simulink model "model5"  (R2022a)
settings: Solver=VariableStepAuto  StartTime=0.0  StopTime=20  MaxStep=0.05  RelTol=1e-3  AbsTol=1e-3  EnableMultiTasking=on
PostLoadFcn:
  | m = 3.600;     % kg
  | k = 400;    % N/m
  | b = 10;      % Ns/m
CloseFcn:
  | try,close(h1_ssc_mass_spring_damper_sl_dbl),end
  | clear h1_ssc_mass_spring_damper_sl_dbl
  | 
  | clear simlog_ssc_mass_spring_damper_sl_dbl
  | clear logsout_ssc_mass_spring_damper_sl_dbl
Description:
  | Double Mass-Spring-Damper in Simulink(R) and Simscape(TM)
settings Model: Creator=The MathWorks, Inc.  LastModifiedBy=whatastarrynight
settings SolverCC: AutoScaleAbsTol=off  AlgebraicLoopSolver=TrustRegion
settings DataIOCC: LimitDataPoints=on  SaveFormat=Array  ReturnWorkspaceOutputs=off  SignalLoggingName=logsout_ssc_mass_spring_damper_sl_dbl
settings OptimizationCC: LifeSpan=inf
settings DebuggingCC: SolverPrmCheckMsg=warning  UnconnectedInputMsg=warning  UnconnectedOutputMsg=warning  UnconnectedLineMsg=warning  AllowSymbolicDim=off  PregeneratedLibrarySubsystemCodeDiagnostic=none  SFUnexpectedBacktrackingDiag=warning  SFNoUnconditionalDefaultTransitionDiag=warning  SFExecutionAtInitializationDiag=none  SFMachineParentedDataDiag=warning  ArithmeticOperatorsInVariantConditions=warning
settings HardwareCC: ProdBitPerPointer=32  ProdBitPerSizeT=32  ProdBitPerPtrDiffT=32  ProdLargestAtomicFloat=None  ProdIntDivRoundTo=Undefined  ProdEndianess=Unspecified  ProdWordSize=32  ProdHWDeviceType=32-bit Generic
settings ModelReferenceCC: PropagateSignalLabelsOutOfModel=off
settings SFSimCC: SimUseLocalCustomCode=off  CustomCodeUndefinedFunction=UseInterfaceOnly
settings RTWCC: RTWUseLocalCustomCode=off  DLArmComputeVersion=19.05
settings CodeAppCC: StateflowObjectComments=on
settings GRTTargetCC: TargetLangStandard=C89/C90 (ANSI)
settings ConfigComp: CovMetricSettings=dw  CovSaveCumulativeToWorkspaceVar=on  CovSaveSingleToWorkspaceVar=on  CovExternalEMLEnable=off  CovSFcnEnable=off
settings SimscapeCC: SimscapeLogType=all  SimscapeLogSimulationStatistics=on  SimscapeLogName=simlog_ssc_mass_spring_damper_sl_dbl  SimscapeLogDataHistory=10000

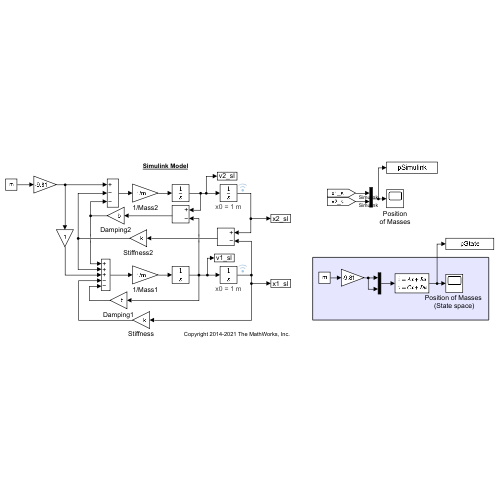
[thumbnail: Simulink's stored preview of the top-level diagram]
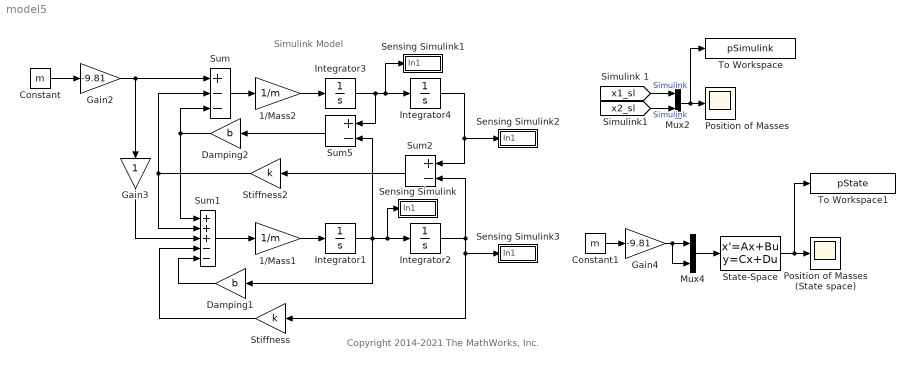
== system model5 ==
  note: Simulink Model
  note: Copyright 2014-2021 The MathWorks, Inc.
  1/Mass1 : Gain  Gain=1/m  SaturateOnIntegerOverflow=on  OutDataTypeStr=Inherit: Same as input  ParamDataTypeStr=Inherit: Same as input
  1/Mass2 : Gain  Gain=1/m  SaturateOnIntegerOverflow=on  OutDataTypeStr=Inherit: Same as input  ParamDataTypeStr=Inherit: Same as input
  Constant : Constant  Value=m
  Constant1 : Constant  Value=m
  Damping1 : Gain  Gain=b  SaturateOnIntegerOverflow=on  OutDataTypeStr=Inherit: Same as input  ParamDataTypeStr=Inherit: Same as input
  Damping2 : Gain  Gain=b  SaturateOnIntegerOverflow=on  OutDataTypeStr=Inherit: Same as input  ParamDataTypeStr=Inherit: Same as input
  Gain2 : Gain  Gain=-9.81
  Gain3 : Gain
  Gain4 : Gain  Gain=-9.81
  Integrator1 : Integrator
  Integrator2 : Integrator  InitialCondition=1
      settings: AttributesFormatString=x0 = %<InitialCondition> m
  Integrator3 : Integrator
  Integrator4 : Integrator  InitialCondition=1
      settings: AttributesFormatString=x0 = %<InitialCondition> m
  Mux2 : Mux  Inputs=2
  Mux4 : Mux  Inputs=2
  Position of Masses : Scope
  Position of Masses (State space) : Scope
  Sensing Simulink : Subsystem
      mask Display: disp('v1_sl')
  Sensing Simulink1 : Subsystem
      mask Display: disp('v2_sl')
  Sensing Simulink2 : Subsystem
      mask Display: disp('x2_sl')
  Sensing Simulink3 : Subsystem
      mask Display: disp('x1_sl')
  State-Space : StateSpace  A=[0,1,0,0;-2*k/m,-2*b/m,k/m,b/m;0,0,0,1;k/m,b/m,-k/m,-b/m]  B=[0,0;1/m,0;0,0;0,1/m]  C=[1,0,0,0;0,0,1,0]  D=[0,0;0,0]  InitialCondition=[1,0,1,0]
  Stiffness : Gain  Gain=k  SaturateOnIntegerOverflow=on  OutDataTypeStr=Inherit: Same as input  ParamDataTypeStr=Inherit: Same as input
  Stiffness2 : Gain  Gain=k  SaturateOnIntegerOverflow=on  OutDataTypeStr=Inherit: Same as input  ParamDataTypeStr=Inherit: Same as input
  Sum : Sum  Inputs=+--  InputSameDT=on  SaturateOnIntegerOverflow=on  OutDataTypeStr=Inherit: Same as first input
  Sum1 : Sum  Inputs=+++--  InputSameDT=on  SaturateOnIntegerOverflow=on  OutDataTypeStr=Inherit: Same as first input
  Sum2 : Sum  Inputs=+-  InputSameDT=on  SaturateOnIntegerOverflow=on  OutDataTypeStr=Inherit: Same as first input
  Sum5 : Sum  Inputs=+-  InputSameDT=on  SaturateOnIntegerOverflow=on  OutDataTypeStr=Inherit: Same as first input
  To Workspace : ToWorkspace  VariableName=pSimulink  SaveFormat=Timeseries  SampleTime=-1
  To Workspace1 : ToWorkspace  VariableName=pState  SaveFormat=Timeseries  SampleTime=-1
  wires:
  1/Mass1/1 -> Integrator1/1
  Sum1/1 -> 1/Mass1/1
  Sum5/1 -> Damping2/1
  Damping2/1 -> Sum1/1, Sum/3
  1/Mass2/1 -> Integrator3/1
  Sum/1 -> 1/Mass2/1
  Integrator4/1 -> Sensing Simulink2/1(In1), Sum2/1
  Integrator3/1 -> Sensing Simulink1/1(In1), Integrator4/1, Sum5/1
  Sum2/1 -> Stiffness2/1
  Stiffness2/1 -> Sum1/2, Sum/2
  Damping1/1 -> Sum1/5
  Stiffness/1 -> Sum1/4
  Integrator1/1 -> Sum5/2, Sensing Simulink/1(In1), Integrator2/1, Damping1/1
  Mux2/1 -> To Workspace/1, Position of Masses/1
  Integrator2/1 -> Stiffness/1, Sensing Simulink3/1(In1), Sum2/2
  Constant/1 -> Gain2/1
  Gain2/1 -> Gain3/1, Sum/1
  Gain3/1 -> Sum1/3
  Constant1/1 -> Gain4/1
  State-Space/1 -> To Workspace1/1, Position of Masses (State space)/1
  Gain4/1 -> Mux4/2, Mux4/1
  Mux4/1 -> State-Space/1
  [x1_sl] -> Mux2/1  "Simulink"
  [x2_sl] -> Mux2/2  "Simulink"

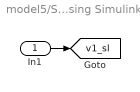
== system model5/Sensing Simulink ==
  In1 : Inport
  tag scope: v1_sl=global
  wires:
  In1/1 -> [v1_sl]

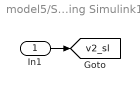
== system model5/Sensing Simulink1 ==
  In1 : Inport
  tag scope: v2_sl=global
  wires:
  In1/1 -> [v2_sl]

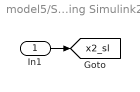
== system model5/Sensing Simulink2 ==
  In1 : Inport
  tag scope: x2_sl=global
  wires:
  In1/1 -> [x2_sl]

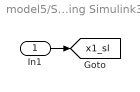
== system model5/Sensing Simulink3 ==
  In1 : Inport
  tag scope: x1_sl=global
  wires:
  In1/1 -> [x1_sl]
